simulink model "Traffic_Light"  (R2021a)
settings: Solver=FixedStepAuto  StartTime=0.0  StopTime=10.0  FixedStep=1  RelTol=1e-3
settings Model: Creator=Osman  LastModifiedBy=Osman

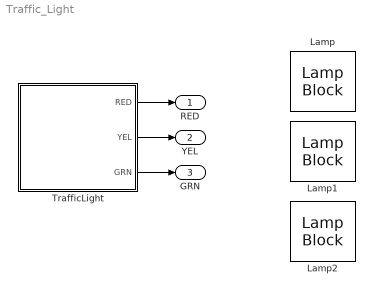
== system Traffic_Light ==
  Lamp : LampBlock
  Lamp1 : LampBlock
  Lamp2 : LampBlock
  TrafficLight : Stateflow chart  TreatAsAtomicUnit=on
  RED : Outport
  YEL : Outport  Port=2
  GRN : Outport  Port=3
  wires:
  TrafficLight/2(YEL) -> YEL/1
  TrafficLight/3(GRN) -> GRN/1
  TrafficLight/1(RED) -> RED/1

== stateflow chart Traffic_Light/TrafficLight ==
  state stop
    entry:
    RED = 1;
    YEL = 0;
    GRN = 0;
  state ready
    entry:
    RED = 0;
    YEL = 1;
    GRN = 0;
  state go
    entry:
    RED = 0;
    YEL = 0;
    GRN = 1;
  (default) -> stop
  go -> stop : after(3,sec)
  stop -> ready : after(3,sec)
  ready -> go : after(1,sec)
  data: RED output uint8; YEL output uint8; GRN output uint8
